simulink model "UAV_Model"  (R2022b)
settings: Solver=VariableStepAuto  StartTime=0.0  StopTime=50  RelTol=1e-3
values from neighbouring files (symbols this model uses):
  d0 = 2.0    (= 2)    [lidar_script.m]
  g = 9.81    [lidar_script.m]
  Ib = diag([1.2416 1.2416 2*1.2416])    [lidar_script.m]
  initori = [0 0 0]    [lidar_script.m]
  initpos = [0 0 -5]    [lidar_script.m]
  initvel = [0 0 0]    [lidar_script.m]
  k_att = 0.5    [lidar_script.m]
  k_rep = 0.5    [lidar_script.m]
  kp = diag([40 40 40])    [lidar_script.m]
  kr = diag([40 40 40])    [lidar_script.m]
  kv = diag([10 10 10])    [lidar_script.m]
  kw = diag([10 10 10])    [lidar_script.m]
  mass = 1.2    [lidar_script.m]
  q_goal = [9 9 -5]    [lidar_script.m]
  Ts = 0.01    [lidar_script.m]
  u0_t = 11.77    [lidar_script.m]
undefined symbols (not defined in the file or in its folder): Lidar, platformUAV
libraries: uavsimlib x6, robotcorelib x4, shareduavrstlib x1, uavalgslib x1
settings Model: VariantFading=off  Creator=The MathWorks, Inc.  LastModifiedBy=stefa
settings DebuggingCC: UnconnectedInputMsg=warning  UnconnectedOutputMsg=warning  UnconnectedLineMsg=warning
settings ModelReferenceCC: EnableRefExpFcnMdlSchedulingChecks=on
settings RTWCC: DLArmComputeVersion=19.05

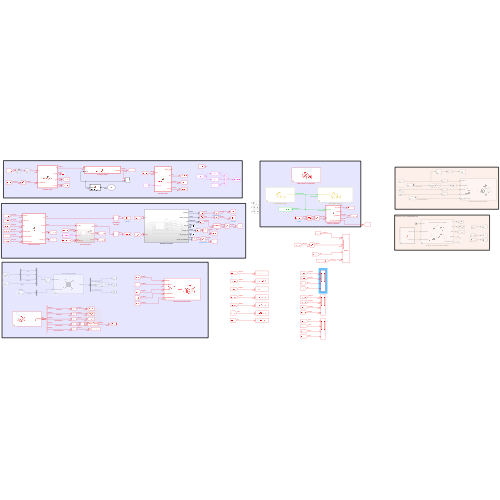
[thumbnail: Simulink's stored preview of the top-level diagram]
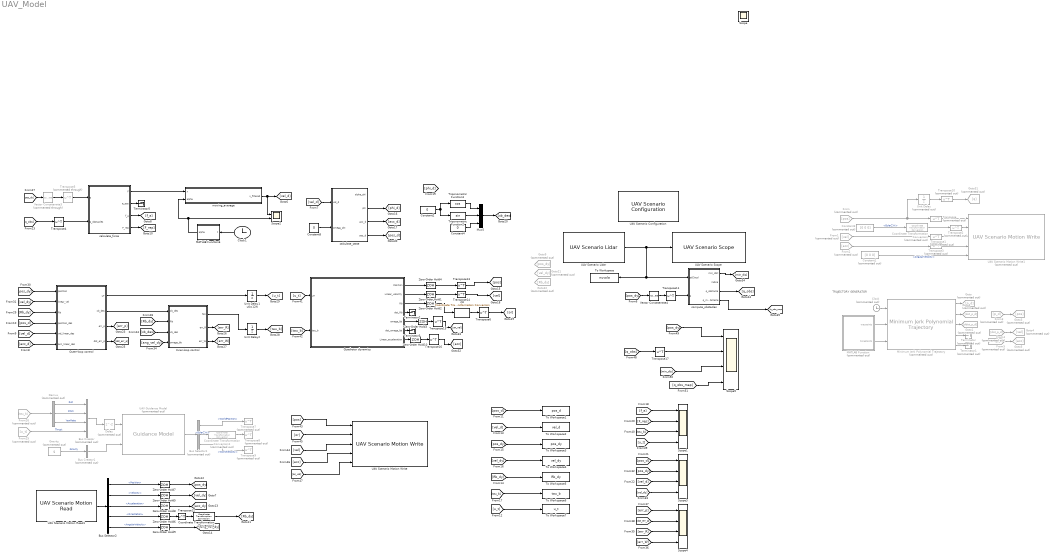
== system UAV_Model ==
  note: TRAJECTORY GENERATOR
  Bus Creator : BusCreator  Commented=on  Inputs=4  OutDataTypeStr=Bus: MultirotorGuidanceControlBus  NonVirtualBus=on
  Bus Creator1 : BusCreator  Commented=on  Inputs=1  OutDataTypeStr=Bus: MultirotorGuidanceEnvironmentBus  NonVirtualBus=on
  Bus Selector1 : BusSelector  Commented=on  OutputSignals=WorldPosition,EulerZYX,WorldVelocity
  Bus Selector2 : BusSelector  OutputSignals=Position,Velocity,Acceleration,Orientation,AngularVelocity
  Clock : Clock  Commented=on
  Clock1 : Clock
  Constant1 : Constant  Commented=on  Value=[0 0 0]
  Constant2 : Constant  Value=0
  Constant3 : Constant  Commented=on  Value=[0 0 0]
  Constant4 : Constant  Value=0
  Constant8 : Constant  Value=0
  Coordinate Transformation Conversion : robotcorelib/Coordinate Transformation Conversion  Commented=on  InputRepresentation=Euler Angles  InputEulerSequence=ZYX  ShowTrVecInputPort=on  OutputRepresentation=Quaternion  OutputEulerSequence=ZYX  ShowTrVecOutputPort=on  SimulateUsing=Interpreted execution
  Coordinate Transformation Conversion1 : robotcorelib/Coordinate Transformation Conversion  Commented=on  InputRepresentation=Euler Angles  InputEulerSequence=ZYX  ShowTrVecInputPort=on  OutputRepresentation=Quaternion  OutputEulerSequence=ZYX  ShowTrVecOutputPort=on  SimulateUsing=Interpreted execution
  Coordinate Transformation Conversion2 : robotcorelib/Coordinate Transformation Conversion  InputRepresentation=Quaternion  InputEulerSequence=ZYX  ShowTrVecInputPort=on  OutputRepresentation=Rotation Matrix  OutputEulerSequence=ZYX  ShowTrVecOutputPort=on  SimulateUsing=Interpreted execution
  Delay : Delay  Commented=on
  Demux : Demux  Commented=on  Outputs=3
  From : From  Commented=on  GotoTag=pos
  From1 : From  Commented=on  GotoTag=vel
  From2 : From  Commented=on  GotoTag=acc
  From25 : From  Commented=on  GotoTag=u_t
  From26 : From  Commented=on  GotoTag=tau_b
  From3 : From  Commented=on  GotoTag=p_d
  From4 : From  Commented=on  GotoTag=dot_p_d
  From5 : From  Commented=on  GotoTag=ddot_p_d
  Goto : Goto  Commented=on  GotoTag=p_d
  Goto1 : Goto  Commented=on  GotoTag=ddot_p_d
  Goto2 : Goto  Commented=on  GotoTag=dot_p_d
  Goto21 : Goto  Commented=on  GotoTag=vel_dy
  Goto22 : Goto  Commented=on  GotoTag=Rb_dy
  Goto3 : Goto  Commented=on  GotoTag=pos
  Goto31 : Goto  Commented=on  GotoTag=q
  Goto4 : Goto  Commented=on  GotoTag=vel
  Goto5 : Goto  Commented=on  GotoTag=acc
  Goto9 : Goto  Commented=on  GotoTag=pos_dy
  Gravity : Constant  Commented=on  Value=g
  Inner-loop control : Subsystem
  MATLAB Function : MATLAB Function  Commented=on  TreatAsAtomicUnit=on
  MATLAB Function6 : MATLAB Function  TreatAsAtomicUnit=on
  Minimum Jerk Polynomial Trajectory : shareduavrstlib/Minimum Jerk Polynomial Trajectory  Commented=on  ShowBCInputPort=off  ShowPolynomialCoefs=off  ShowStatusOutputPort=off  TimeAllocation=off  TimeWeight=100  MinSegmentTime=0.1  MaxSegmentTime=1  MaxIteration=1500  MaxTime=10  SimulateUsing=Interpreted execution
      settings: LibrarySourceBlock=uavalgslib/Minimum Jerk Polynomial Trajectory
  Mux5 : Mux  Inputs=3
  Outer-loop control : MATLAB Function  TreatAsAtomicUnit=on
  Quadrotor dynamics : Subsystem
  Scope{1,3..5} (4 alike) : Scope  NumInputPorts=4
  Scope2 : Scope  NumInputPorts=2
  Terminator : Terminator  Commented=on
  Terminator1 : Terminator  Commented=on
  Terminator2 : Terminator
  Terminator3 : Terminator
  Terminator5 : Terminator
  To Workspace : ToWorkspace  VariableName=nuvola  SaveFormat=Timeseries  SampleTime=-1
  To Workspace1 : ToWorkspace  VariableName=pos_d  SaveFormat=Timeseries  SampleTime=-1
  To Workspace2 : ToWorkspace  VariableName=vel_d  SaveFormat=Timeseries  SampleTime=-1
  To Workspace3 : ToWorkspace  VariableName=pos_dy  SaveFormat=Timeseries  SampleTime=-1
  To Workspace4 : ToWorkspace  VariableName=vel_dy  SaveFormat=Timeseries  SampleTime=-1
  To Workspace5 : ToWorkspace  VariableName=Rb_dy  SaveFormat=Timeseries  SampleTime=-1
  To Workspace6 : ToWorkspace  VariableName=tau_b  SaveFormat=Timeseries  SampleTime=-1
  To Workspace7 : ToWorkspace  VariableName=u_t  SaveFormat=Timeseries  SampleTime=-1
  Transpose{,1..3,7..10} (8 alike) : Math  Commented=on  Operator=transpose
  Transpose{4,6,11..17} (9 alike) : Math  Operator=transpose
  Transpose5 : Math  Commented=through  Operator=transpose
  Trigonometric Function2 : Trigonometry
  Trigonometric Function3 : Trigonometry  Operator=cos
  UAV Guidance Model : uavalgslib/Guidance Model  Commented=on  ModelType=MultirotorGuidance  SpecifiedDataType=double  SimulateUsing=Interpreted execution  InitialWorldPositionMultirotor=initpos'  InitialWorldVelocityMultirotor=initvel'  InitialEulerZYXMultirotor=initori'  InitialBodyAngularRateRPYMultirotor=[0; 0; 0]  InitialThrustMultirotor=u0_t  InitialNorthFixedWing=0  InitialEastFixedWing=0  InitialHeightFixedWing=0  InitialAirSpeedFixedWing=0  InitialHeadingAngleFixedWing=0  InitialFlightPathAngleFixedWing=0  InitialRollAngleFixedWing=0  InitialRollAngleRateFixedWing=0  PDRollMultirotor=[1 1]  PDPitchMultirotor=[1 1]  PYawRateMultirotor=1  PThrustMultirotor=1  MassMultirotor=mass  PHeightFixedWing=3.9  PHeadingAngleFixedWing=3.9  PFlightPathAngleFixedWing=39  PDRollFixedWing=[3402.97, 116.67]  PAirSpeedFixedWing=1  FlightPathAngleLimitsFixedWing=[-pi/2, pi/2]  StateBusName='MultirotorGuidanceStateBus'  ControlBusName='MultirotorGuidanceControlBus'  EnvironmentBusName='MultirotorGuidanceEnvironmentBus'  DataType=double
  UAV Scenario Configuration : uavsimlib/UAV Scenario Configuration  Priority=-1  UAVScenarioObject=scene  SampleTime=0.01  UpdateParam=true  SensorMotionBusName='SensorMotionBus'  PlatformMotionBusName='PlatformMotionBus'  ScenarioMotionBusName='ScenarioMotionBus'  ScenarioMotionSignalName='ScenarioMotions'
  UAV Scenario Lidar : uavsimlib/UAV Scenario Lidar  Priority=1  SensorName=platformUAV/Lidar  MaxRange=10  RangeAccuracy=0.02  AzimuthLimits=[ -180, 180 ]  AzimuthResolution=0.16  ElevationLimits=[ -20, 20 ]  ElevationResolution=1.25  HasNoise=off  HasOrganizedOutput=on  SampleTime=0.1
  UAV Scenario Motion Read1 : uavsimlib/UAV Scenario Motion Read  Priority=1  EntityName='platformUAV'  ReferenceFrame=NED
  UAV Scenario Motion Write : uavsimlib/UAV Scenario Motion Write  Priority=0  PlatName='platformUAV'  ReferenceFrame=NED
  UAV Scenario Motion Write1 : uavsimlib/UAV Scenario Motion Write  Priority=0  Commented=on  PlatName='platformUAV'  ReferenceFrame=NED
  UAV Scenario Scope : uavsimlib/UAV Scenario Scope  Priority=1  SensorNameTable={ 'platformUAV/Lidar', 'on' }  SampleTime=0.1
  Unit Delay : UnitDelay  Commented=on  InitialCondition=initpos  SampleTime=Ts  HasFrameUpgradeWarning=on
  Unit Delay1 u0=12N : UnitDelay  InitialCondition=u0_t  SampleTime=Ts
  Unit Delay2 : UnitDelay  InitialCondition=[0 0 0]  SampleTime=Ts
  Vector Concatenate3 : Concatenate  Commented=through  NumInputs=1  Mode=Multidimensional array
  Vector Concatenate4 : Concatenate  NumInputs=1  Mode=Multidimensional array
  Zero-Order Hold{1..2,4,10} (4 alike) : ZeroOrderHold  SampleTime=0.01
  Zero-Order Hold{3,5..9} (6 alike) : ZeroOrderHold  SampleTime=Ts
  calculate_force : MATLAB Function  TreatAsAtomicUnit=on
  calculate_state : MATLAB Function  TreatAsAtomicUnit=on
  compute_obstacles : MATLAB Function  TreatAsAtomicUnit=on
  ctc : robotcorelib/Coordinate Transformation Conversion  InputRepresentation=Rotation Matrix  InputEulerSequence=ZYX  ShowTrVecInputPort=on  OutputRepresentation=Quaternion  OutputEulerSequence=ZYX  ShowTrVecOutputPort=on  SimulateUsing=Interpreted execution
  moving_average : MATLAB Function  TreatAsAtomicUnit=on
  Scope : Scope
  wires:
  UAV Scenario Lidar/1 -> To Workspace/1, compute_obstacles/1(ptCloud), UAV Scenario Scope/1
  Transpose3/1 -> UAV Scenario Motion Write1/4
  Constant1/1 -> UAV Scenario Motion Write1/5  "<AngularVelocity>"
  Bus Creator/1 -> Delay/1
  Demux/1 -> Bus Creator/1  "Roll"
  From25/1 -> Bus Creator/4  "Thrust"
  Demux/2 -> Bus Creator/2  "Pitch"
  Demux/3 -> Bus Creator/3  "YawRate"
  Gravity/1 -> Bus Creator1/1  "Gravity"
  Transpose1/1 -> UAV Scenario Motion Write1/3
  Coordinate Transformation Conversion/1 -> Transpose2/1
  Transpose2/1 -> UAV Scenario Motion Write1/2
  UAV Guidance Model/1 -> Bus Selector1/1
  Delay/1 -> UAV Guidance Model/1
  Bus Creator1/1 -> UAV Guidance Model/2
  From2/1 -> Transpose3/1
  From1/1 -> Transpose1/1
  From/1 -> Unit Delay/1, Transpose/1
  Constant3/1 -> Coordinate Transformation Conversion/1  "<EulerZYX>"
  Transpose11/1 -> compute_obstacles/2(q)
  compute_obstacles/3(q_obstacle) -> [q_obs]
  Trigonometric Function3/1 -> Mux5/1
  Constant4/1 -> Mux5/3
  Constant2/1 -> Trigonometric Function2/1, Trigonometric Function3/1
  Trigonometric Function2/1 -> Mux5/2
  Clock1/1 -> MATLAB Function6/1(t)
  Constant8/1 -> calculate_state/2(omega_phi)
  calculate_state/2(phi) -> [phi_d]
  moving_average/1(x_filtered) -> Scope2/1, [vel_d]
  MATLAB Function6/1(alpha) -> moving_average/2(alpha), Scope2/2
  Minimum Jerk Polynomial Trajectory/3 -> Goto1/1
  Minimum Jerk Polynomial Trajectory/4 -> Terminator/1
  From3/1 -> Goto3/1
  Minimum Jerk Polynomial Trajectory/5 -> Terminator1/1
  Minimum Jerk Polynomial Trajectory/2 -> Goto2/1
  MATLAB Function/1(waypoints) -> Minimum Jerk Polynomial Trajectory/2
  Minimum Jerk Polynomial Trajectory/1 -> Goto/1
  From4/1 -> Goto4/1
  MATLAB Function/2(timePoints) -> Minimum Jerk Polynomial Trajectory/3
  From5/1 -> Goto5/1
  Clock/1 -> Minimum Jerk Polynomial Trajectory/1
  [q_obs] -> Transpose4/1
  Transpose4/1 -> calculate_force/2(q_obstacles)
  calculate_force/1(F) -> moving_average/1(x)
  [pos_dy] -> Vector Concatenate3/1
  Transpose/1 -> UAV Scenario Motion Write1/1
  Quadrotor dynamics/1(Position) -> Zero-Order Hold4/1
  Outer-loop control/2(zb_des) -> Inner-loop control/1(zb_des)
  Zero-Order Hold4/1 -> Transpose13/1
  Quadrotor dynamics/6(dot_omega_bb) -> Terminator3/1
  Quadrotor dynamics/5(omega_bb) -> Zero-Order Hold3/1
  [xb_des] -> Inner-loop control/3(xb_des)
  [vel_d] -> Outer-loop control/5(vel_linear_des)
  Quadrotor dynamics/4(dot_Rb) -> Terminator2/1
  Zero-Order Hold2/1 -> ctc/1
  [acc_d] -> Outer-loop control/6(acc_linear_des)
  Inner-loop control/2(err_R) -> [err_R]
  Zero-Order Hold1/1 -> Transpose14/1
  Inner-loop control/3(err_W) -> [err_W]
  Inner-loop control/1(tau) -> Unit Delay2/1
  Unit Delay1 u0=12N/1 -> [u_t]
  Quadrotor dynamics/2(Linear_velocity) -> Zero-Order Hold1/1
  Unit Delay2/1 -> [tau_b]
  Outer-loop control/3(err_p) -> [err_p]
  Outer-loop control/1(uT) -> Unit Delay1 u0=12N/1
  [pos_d] -> Outer-loop control/4(position_des)
  Outer-loop control/4(dot_err_p) -> [dot_err_p]
  Quadrotor dynamics/3(Rb) -> Zero-Order Hold2/1
  ctc/1 -> Transpose6/1
  Bus Selector1/2 -> Coordinate Transformation Conversion1/1  "<EulerZYX>"
  From26/1 -> Demux/1
  [pos] -> UAV Scenario Motion Write/1
  [or] -> UAV Scenario Motion Write/2
  [vel] -> UAV Scenario Motion Write/3
  Unit Delay/1 -> Transpose10/1
  Transpose10/1 -> Goto31/1
  Transpose6/1 -> [or]
  [Rb_dy] -> Inner-loop control/2(Rb)
  [Rb_dy] -> Outer-loop control/3(Rb)
  [pos_dy] -> Outer-loop control/1(position)
  [vel_dy] -> Outer-loop control/2(linear_vel)
  Vector Concatenate3/1 -> Transpose5/1
  Transpose5/1 -> calculate_force/1(q)
  [pos_dy] -> Vector Concatenate4/1
  Vector Concatenate4/1 -> Transpose11/1
  calculate_state/3(acc_d) -> [acc_d]
  calculate_state/4(pos_d) -> [pos_d]
  [vel_d] -> calculate_state/1(vel_d)
  calculate_force/4(F_rep) -> [F_rep]
  calculate_force/3(f_a) -> [f_a]
  calculate_force/2(e_pos) -> Terminator5/1
  [pos_d] -> To Workspace1/1
  [vel_d] -> To Workspace2/1
  [pos_dy] -> To Workspace3/1
  [vel_dy] -> To Workspace4/1
  [Rb_dy] -> To Workspace5/1
  [tau_b] -> To Workspace6/1
  [u_t] -> To Workspace7/1
  [F_rep] -> Scope1/2
  [f_a] -> Scope1/1
  [vel_dy] -> Scope3/4
  [vel_d] -> Scope3/3
  [pos_dy] -> Scope3/2
  [pos_d] -> Scope3/1
  Bus Selector2/4 -> Zero-Order Hold6/1  "<Orientation>"
  UAV Scenario Motion Read1/1 -> Bus Selector2/1
  Bus Selector2/1 -> Zero-Order Hold7/1  "<Position>"
  Bus Selector2/5 -> Zero-Order Hold9/1  "<AngularVelocity>"
  Bus Selector2/2 -> Zero-Order Hold5/1  "<Velocity>"
  Bus Selector2/3 -> Zero-Order Hold8/1  "<Acceleration>"
  Zero-Order Hold7/1 -> [pos_dy]
  Zero-Order Hold5/1 -> [vel_dy]
  Zero-Order Hold6/1 -> Transpose12/1
  Zero-Order Hold8/1 -> [acc_dy]
  Zero-Order Hold9/1 -> [ang_vel_dy]
  Coordinate Transformation Conversion2/1 -> [Rb_dy]
  Transpose12/1 -> Coordinate Transformation Conversion2/1
  [ang_vel_dy] -> Inner-loop control/4(omega_bb)
  [u_t] -> Scope1/4
  Mux5/1 -> [xb_des]
  [err_p] -> Scope4/1
  [dot_err_p] -> Scope4/2
  [err_R] -> Scope4/3
  [err_W] -> Scope4/4
  [tau_b] -> Scope1/3
  [u_t] -> Quadrotor dynamics/1(uT)
  [tau_b] -> Quadrotor dynamics/2(tau_b)
  Transpose13/1 -> [pos]
  Transpose14/1 -> [vel]
  Bus Selector1/1 -> Transpose7/1  "<WorldPosition>"
  Coordinate Transformation Conversion1/1 -> Transpose8/1
  Bus Selector1/3 -> Transpose9/1  "<WorldVelocity>"
  Transpose16/1 -> [acc]
  Zero-Order Hold10/1 -> Transpose16/1
  Quadrotor dynamics/7(Linear_acceleration) -> Zero-Order Hold10/1
  [acc] -> UAV Scenario Motion Write/4
  Zero-Order Hold3/1 -> Transpose15/1
  Transpose15/1 -> [an_vel]
  [an_vel] -> UAV Scenario Motion Write/5
  [pos_dy] -> Scope5/1
  [q_obs] -> Transpose17/1
  [min_dis] -> Scope5/3
  Transpose17/1 -> Scope5/2
  compute_obstacles/1(min_dist) -> [min_dis]
  compute_obstacles/4(q_map_obstacle) -> [q_obs_map]
  [q_obs_map] -> Scope5/4

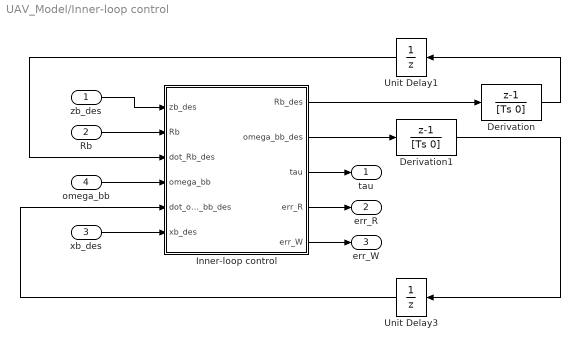
== system UAV_Model/Inner-loop control ==
  zb_des : Inport
  Rb : Inport  Port=2
  xb_des : Inport  Port=3
  omega_bb : Inport  Port=4
  Derivation : DiscreteTransferFcn  Numerator=[1 -1]  Denominator=[Ts 0]  InitialStates=[1 0 0;0 1 0;0 0 1]  SampleTime=Ts
  Derivation1 : DiscreteTransferFcn  Numerator=[1 -1]  Denominator=[Ts 0]  InitialStates=[0 0 0]  SampleTime=Ts
  Inner-loop control : MATLAB Function  TreatAsAtomicUnit=on
  Unit Delay1 : UnitDelay  InitialCondition=eul2rotm(initori)  SampleTime=Ts
  Unit Delay3 : UnitDelay  InitialCondition=[0 0 0]  SampleTime=Ts
  tau : Outport
  err_R : Outport  Port=2
  err_W : Outport  Port=3
  wires:
  Derivation1/1 -> Unit Delay3/1
  Unit Delay3/1 -> Inner-loop control/5(dot_omega_bb_des)
  Inner-loop control/5(err_W) -> err_W/1
  Inner-loop control/3(tau) -> tau/1
  Derivation/1 -> Unit Delay1/1
  Inner-loop control/2(omega_bb_des) -> Derivation1/1
  Inner-loop control/1(Rb_des) -> Derivation/1
  Inner-loop control/4(err_R) -> err_R/1
  zb_des/1 -> Inner-loop control/1(zb_des)
  xb_des/1 -> Inner-loop control/6(xb_des)
  Unit Delay1/1 -> Inner-loop control/3(dot_Rb_des)
  omega_bb/1 -> Inner-loop control/4(omega_bb)
  Rb/1 -> Inner-loop control/2(Rb)

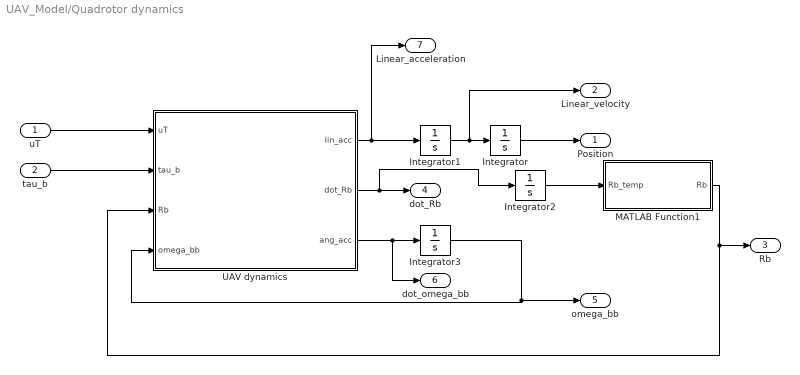
== system UAV_Model/Quadrotor dynamics ==
  uT : Inport
  tau_b : Inport  Port=2
  Integrator : Integrator  InitialCondition=initpos
  Integrator1 : Integrator  InitialCondition=initvel
  Integrator2 : Integrator  InitialCondition=eul2rotm(initori)
  Integrator3 : Integrator  InitialCondition=[0 0 0]
  MATLAB Function1 : MATLAB Function  TreatAsAtomicUnit=on
  UAV dynamics : MATLAB Function  TreatAsAtomicUnit=on
  Position : Outport
  Linear_velocity : Outport  Port=2
  Rb : Outport  Port=3
  dot_Rb : Outport  Port=4
  omega_bb : Outport  Port=5
  dot_omega_bb : Outport  Port=6
  Linear_acceleration : Outport  Port=7
  wires:
  tau_b/1 -> UAV dynamics/2(tau_b)
  Integrator/1 -> Position/1
  UAV dynamics/3(ang_acc) -> dot_omega_bb/1, Integrator3/1
  UAV dynamics/1(lin_acc) -> Integrator1/1, Linear_acceleration/1
  uT/1 -> UAV dynamics/1(uT)
  Integrator1/1 -> Linear_velocity/1, Integrator/1
  Integrator3/1 -> UAV dynamics/4(omega_bb), omega_bb/1
  UAV dynamics/2(dot_Rb) -> Integrator2/1, dot_Rb/1
  MATLAB Function1/1(Rb) -> Rb/1, UAV dynamics/3(Rb)
  Integrator2/1 -> MATLAB Function1/1(Rb_temp)

== matlab function UAV_Model/moving_average ==
  settings: updateMethod=DISCRETE
  data: x input; x_filtered output; alpha input
function x_filtered = exponential_moving_average_vector(x, alpha)
    % Funzione per calcolare la media mobile esponenziale di un vettore colonna 3x1.
    % x: vettore colonna di ingresso 3x1
    % alpha: fattore di smorzamento (0 < alpha < 1)
    % x_filtered: vettore colonna filtrato 3x1
    
%E' lo stesso filtro che abbiamo fatto con Manfredi, la differenza è che
%alpha è tempo variante, varia in funzione esponenziale con il tempo. Se
%allontano l ostacolo nn ho problemi, tanto la Fmax dipende dai
%coefficienti, ma se vario i coefficienti posso dover ritararre il filtro(E' stato inserito per diminuire la trust iniziale)

    % Verifica che l'input x sia un vettore colonna 3x1
    if ~isequal(size(x), [1, 3])
        error('L''input x deve essere un vettore colonna 3x1.');
    end
    
    % Inizializza la variabile persistente
    persistent x_filtered_prev
    
    % Se è la prima chiamata, inizializza la variabile persistente
    if isempty(x_filtered_prev)
        x_filtered_prev = [0 0 0];
    end
    
    % Applica il filtro a media mobile esponenziale elemento per elemento
    x_filtered = (1 - alpha) * x_filtered_prev + alpha * x;
    
    % Aggiorna la variabile persistente
    x_filtered_prev = x_filtered;
end

== matlab function UAV_Model/calculate_force ==
  data: q input; F output; q_obstacles input; q_goal parameter; e_pos output; f_a output; F_rep output; k_att parameter; k_rep parameter; d0 parameter
function [F, e_pos, f_a, F_rep]  = calculate_force(q, q_obstacles, q_goal, k_att, k_rep, d0)
% Funzione per calcolare la forza totale F(q) utilizzando il metodo dei potenziali artificiali
% 
% Inputs:
%   q - Posizione attuale del UAV (3x1 vettore)
%   q_goal - Posizione del goal (3x1 vettore)
%   q_obstacles - Posizioni degli ostacoli (3xn matrice, dove n è il numero di ostacoli)
%   k_att - Coefficiente di attrazione (scalare)
%   k_rep - Coefficiente di repulsione (scalare)
%   d0 - Distanza di influenza degli ostacoli (scalare)
% 
% Output:
%   F - Forza totale (3x1 vettore)

e_pos = q_goal-q;

if(norm(e_pos)<1)
    f_a = k_att * e_pos;
else
    f_a = k_att * e_pos/norm(e_pos);
end
gamma=3;

 % Inizializza la forza repulsiva
F_rep = zeros(1, 3);

q_obs = q_obstacles;
dist = norm(q - q_obs);

if dist <= d0
    eta_q = dist;
    eta_q0 = d0;
    grad_eta_q = (q - q_obs) / dist;
    
    F_rep = F_rep + (k_rep/(eta_q^2))*(1/eta_q - 1/eta_q0)^(gamma-1) * grad_eta_q;
end

F = f_a + F_rep;

% Calcola la forza repulsiva per ciascun ostacolo
% for i = 1:size(q_obstacles, 1)
%     q_obs = q_obstacles(i,:);
%     dist = norm(q - q_obs);
%     
%     if dist <= d0
%         eta_q = dist;
%         eta_q0 = d0;
%         grad_eta_q = (q - q_obs) / dist;
%         
%         F_rep = F_rep + (k_rep/(eta_q^2))*(1/eta_q - 1/eta_q0)^(gamma-1) * grad_eta_q;
%     end
% end
% F = f_a + F_rep;

end

== matlab function UAV_Model/MATLAB Function6 ==
  data: t input; alpha output
function alpha = calculate_alpha(t)
    % Calcola il valore di alpha in base all'istante temporale t
    
    % Define initial and final alpha values
    alpha_initial = 0.0000005;
    alpha_final = 0.5;
    
    % Define the time duration over which alpha should reach final value
    time_to_increase = 10;  % Increase alpha over 10 seconds
    alpha = alpha_initial * (100*t / 2)^2;
    % Calculate alpha based on a combination of slow start and faster growth
%     if t <= 2  % Slow start for the first 2 seconds
%         alpha = alpha_initial * (t / 2)^2;  % Quadratic ramp up
%     else
%         alpha = alpha_initial + (alpha_final - alpha_initial) * ((t - 2) / (time_to_increase - 2));
%     end
    
    % Ensure alpha is within bounds
    alpha = max(min(alpha, alpha_final), alpha_initial);
end

== matlab function UAV_Model/calculate_state ==
  settings: updateMethod=DISCRETE
  data: alpha_phi output; vel_d input; omega_phi input; phi output; acc_d output; pos_d output; initpos parameter; initvel parameter
function [alpha_phi, phi, acc_d, pos_d] = calculate_state(vel_d, omega_phi, initpos, initvel)
    % Calcola le posizioni e le accelerazioni a partire dalle velocità
    % Inizializza le variabili persistenti
    persistent x_prev y_prev z_prev phi_prev
    persistent v_x_prev v_y_prev v_z_prev omega_phi_prev

    Ts = 0.01;
    dt = Ts;

    % Se è la prima chiamata, inizializza le variabili persistenti
    if isempty(x_prev)
        x_prev = initpos(1);
        y_prev = initpos(2);
        z_prev = initpos(3);
        phi_prev = 0;
        v_x_prev = initvel(1);
        v_y_prev = initvel(2);
        v_z_prev = initvel(3);
        omega_phi_prev = 0;
    end

    % Associo le velocità desiderate 
    v_x = vel_d(1);
    v_y = vel_d(2);
    v_z = vel_d(3);
    
    % Calcola le posizioni integrando le velocità
    x = x_prev + v_x * dt;
    y = y_prev + v_y * dt;
    z = z_prev + v_z * dt;
    phi = phi_prev + omega_phi * dt;
    
    % Calcola le accelerazioni derivando le velocità
    a_x = (v_x - v_x_prev) / dt;
    a_y = (v_y - v_y_prev) / dt;
    a_z = (v_z - v_z_prev) / dt;
    alpha_phi = (omega_phi - omega_phi_prev) / dt;
    
    % Sistema gli output
    pos_d = [x; y; z];
    acc_d = [a_x; a_y; a_z];

    % Aggiorna le variabili persistenti
    x_prev = x;
    y_prev = y;
    z_prev = z;
    phi_prev = phi;
    v_x_prev = v_x;
    v_y_prev = v_y;
    v_z_prev = v_z;
    omega_phi_prev = omega_phi;
end

== matlab function UAV_Model/compute_obstacles ==
  data: ptCloud input; min_dist output; q input; indice output; q_obstacle output; q_map_obstacle output
function [min_dist,indice, q_obstacle,q_map_obstacle] = fcn(ptCloud, q)

drone = q;

dim = size(ptCloud);
row = dim(1);   % 32
col = dim(2);   % 2250

q_nuvola = ptCloud;
q_obs_map=ptCloud;

distanze = zeros(row,col);

for i = 1:row

    for j = 1:col
        
        punto = [ptCloud(i,j,1); ptCloud(i,j,2); ptCloud(i,j,3)];

        for k = 1:3
            q_nuvola(i,j,k) = punto(k) - drone(k);
            q_obs_map(i,j,k) = punto(k);
        end
    
        distanze(i,j) = norm([q_nuvola(i,j,1); q_nuvola(i,j,2); q_nuvola(i,j,3)]);

    end

end

% punto più vicino al drone

[min_dist,indice] = min(distanze,[],'all');

[r, c] = ind2sub(size(distanze),indice);

q_obstacle = [q_nuvola(r,c,1); q_nuvola(r,c,2); q_nuvola(r,c,3)];
q_map_obstacle = [q_obs_map(r,c,1); q_obs_map(r,c,2); q_obs_map(r,c,3)];

== matlab function UAV_Model/MATLAB Function ==
  data: waypoints output; timePoints output
function [waypoints,timePoints] = fcn()


waypoints = [0 3 6 10;
             0 3 6 10;
             -5 -5 -5 -5];
timePoints = [0 3 6 9];

% questo attraversa un ostacolo
% waypoints = [0 3.5 7 10;
%              0 3.5 7 10;
%              -5 -6 -7 -8];
% timePoints = [0 3 6 9];

== matlab function UAV_Model/Outer-loop control ==
  data: position input size=3; uT output size=1; linear_vel input size=3; Rb input size=[3,3]; zb_des output size=3; mass parameter size=1; position_des input size=3; vel_linear_des input size=3; acc_linear_des input size=3; err_p output size=3; dot_err_p output size=3; kp parameter; kv parameter; g parameter
function [uT, zb_des, err_p, dot_err_p] = fcn(position, linear_vel, Rb, mass, ...
    position_des, vel_linear_des, acc_linear_des, kp, kv, g)

%% WRITE HERE THE OUTER-LOOP CONTROL
% position: linear position measure
% linear_vel: linear velocity measure
% Rb: current rotation matrix
% mass: mass of the UAV
% positon_des: desired linear position from the planner
% vel_linear_des: desired linear velocity from the planner
% acc_linear_des: desired linear acceleration from the planner
% ---
% uT: commanded total thrust
% zb_des: desired z-axis of the body frame
% err_p: position error
% dot_err_p: time derivative of the positon error

%% OUTER-LOOP CONTROL

err_p = position - position_des;
dot_err_p = linear_vel - vel_linear_des;


% NON SO COME CHIAMARLA se avete fantasia diamogli un nome decente
num = -kp * err_p - kv * dot_err_p - mass * g * [0; 0; 1] + mass * acc_linear_des;

uT = ((-num')* Rb * [0; 0; 1]);  

zb_des = - num / norm(num);

== matlab function UAV_Model/Inner-loop control/Inner-loop control ==
  data: Rb_des output size=[3,3]; omega_bb_des output size=3; tau output size=3; zb_des input size=3; Rb input size=[3,3]; dot_Rb_des input size=[3,3]; omega_bb input size=3; dot_omega_bb_des input size=3; xb_des input size=3; Ib parameter size=[3,3]; err_R output size=3; err_W output size=3; kw parameter; kr parameter
function [Rb_des,omega_bb_des,tau,err_R,err_W] = fcn(zb_des,Rb,dot_Rb_des,omega_bb,dot_omega_bb_des,xb_des,Ib, kw, kr)

%% WRITE HERE THE INNER-LOOP CONTROL
% zb_des: desired z-axis of the body frame
% Rb: current rotation matrix
% dot_Rb_des: time-derivative of the desired rotation matrix
% omega_bb: current angular velocity expressed in the body frame
% dot_omega_bb_des: desired angular acceleration expressed in the body
% frame
% xb_des: desired x-axis of the body frame form the planner
% Ib: inertia matrix of the UAV with respect to the body frame
% ---
% Rb_des: desired rotation matrix
% omega_bb_des: desired angular velocity expressed in the body frame (given
% below as a hint)
% tau: commanded control torque
% err_R: rotational error in SO(3)
% err_W: angular velocity error in SO(3)

yb_des=( skew(zb_des) * xb_des) / norm( ( skew(zb_des) * xb_des) );

Rb_des=[skew(yb_des)*zb_des yb_des zb_des];

err_R= 1/2 * wedge( (Rb_des') * Rb - (Rb') * Rb_des);

omega_bb_des = wedge(Rb_des'*dot_Rb_des);

err_W=omega_bb - (Rb') * Rb_des * omega_bb_des; 

tau=-kr * err_R - kw * err_W + skew(omega_bb) * Ib * omega_bb - Ib * (skew(omega_bb) * (Rb') * Rb_des * omega_bb_des - (Rb') * Rb_des * dot_omega_bb_des);
end

function S = skew(v)
if(numel(v)~= 1)
S= [0 -v(3) v(2); 
    v(3) 0 -v(1);
    -v(2) v(1) 0];
else
S= zeros(3);
end
end

function v = wedge(S)
v1 = S(3,2);
v2 = S(1,3);
v3 = S(2,1);
v = [v1 v2 v3]';
end

== matlab function UAV_Model/Quadrotor dynamics/MATLAB Function1 ==
  data: Rb_temp input; Rb output
function Rb = fcn(Rb_temp)
    [U,S,V] = svd(Rb_temp);
    sigma = det(U*V');
    S_ = diag([1 1 sigma]);

    Rb = U*S_*V';
end

== matlab function UAV_Model/Quadrotor dynamics/UAV dynamics ==
  data: uT input size=1; tau_b input size=3; lin_acc output size=3; Rb input size=[3,3]; omega_bb input size=3; dot_Rb output size=[3,3]; ang_acc output size=3; mass parameter size=1; Ib parameter size=[3,3]
function [lin_acc, dot_Rb, ang_acc] = fcn(uT,tau_b,Rb,omega_bb,mass, Ib)

lin_acc = 9.81*[0 0 1]'-(uT/mass)*Rb*[0 0 1]';
dot_Rb = Rb*skew(omega_bb);
ang_acc = inv(Ib)*(-skew(omega_bb)*Ib*omega_bb + tau_b);

end

function S = skew(v)
if(numel(v)~= 1)
S= [0 -v(3) v(2); 
    v(3) 0 -v(1);
    -v(2) v(1) 0];
else
S= zeros(3);
end
end
